simulink model "Subsystem1"  (R2020a)
settings: Solver=VariableStepAuto  StartTime=0.0  StopTime=10.0  RelTol=1e-3
model workspace (MAT data in the model file):
  m = Simulink.Parameter
  m.Value = 1000
  m.DataType = 'auto'
  m.Dimensions = [1 1]
settings Model: Creator=anjal  LastModifiedBy=anjal
settings DataIOCC: SaveOutput=off  SaveTime=off

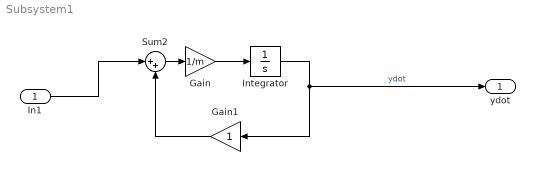
== system Subsystem1 ==
  In1 : Inport  OutDataTypeStr=double  PortDimensions=1  SampleTime=0
  Gain : Gain  Gain=1/m
  Gain1 : Gain
  Integrator : Integrator
  Sum2 : Sum  Inputs=|++
  ydot : Outport  OutDataTypeStr=double  PortDimensions=1  SampleTime=0
  wires:
  Gain1/1 -> Sum2/2
  Integrator/1 -> Gain1/1, ydot/1  "ydot"
  Gain/1 -> Integrator/1
  Sum2/1 -> Gain/1
  In1/1 -> Sum2/1
